simulink model "AirFlow"  (R2015a)
settings: Solver=ode45  StartTime=0.0  StopTime=10.0  RelTol=1e-3
settings Model: Creator=laragoxhaj  LastModifiedBy=laragoxhaj

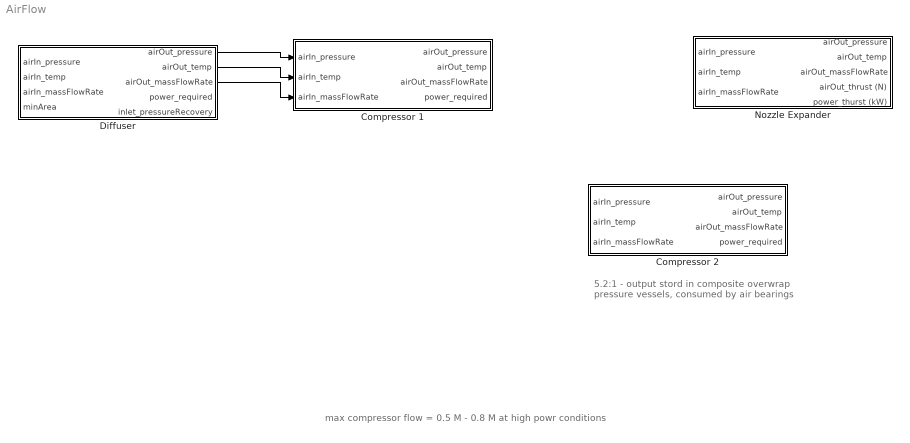
== system AirFlow ==
  note: max compressor flow = 0.5 M - 0.8 M at high powr conditions
  note: 5.2:1 - output stord in composite overwrap
      | pressure vessels, consumed by air bearings
  Compressor 1 : Subsystem
  Compressor 2 : Subsystem
  Diffuser : Subsystem
  Nozzle Expander : Subsystem
  wires:
  Diffuser/1(airOut_pressure) -> Compressor 1/1(airIn_pressure)
  Diffuser/2(airOut_temp) -> Compressor 1/2(airIn_temp)
  Diffuser/3(airOut_massFlowRate) -> Compressor 1/3(airIn_massFlowRate)

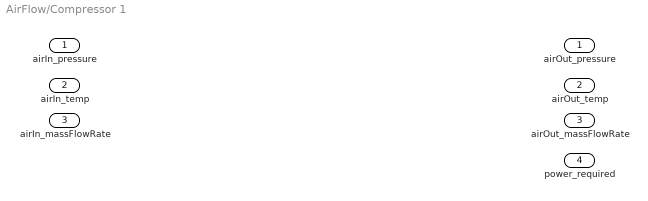
== system AirFlow/Compressor 1 ==
  airIn_pressure : Inport
  airIn_temp : Inport  Port=2
  airIn_massFlowRate : Inport  Port=3
  airOut_pressure : Outport
  airOut_temp : Outport  Port=2
  airOut_massFlowRate : Outport  Port=3
  power_required : Outport  Port=4

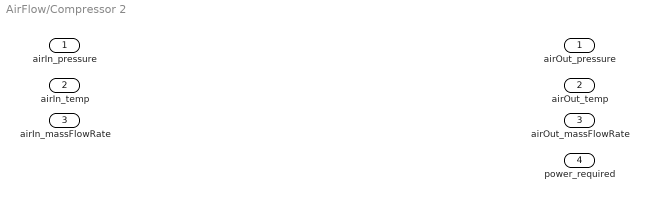
== system AirFlow/Compressor 2 ==
  airIn_pressure : Inport
  airIn_temp : Inport  Port=2
  airIn_massFlowRate : Inport  Port=3
  airOut_pressure : Outport
  airOut_temp : Outport  Port=2
  airOut_massFlowRate : Outport  Port=3
  power_required : Outport  Port=4

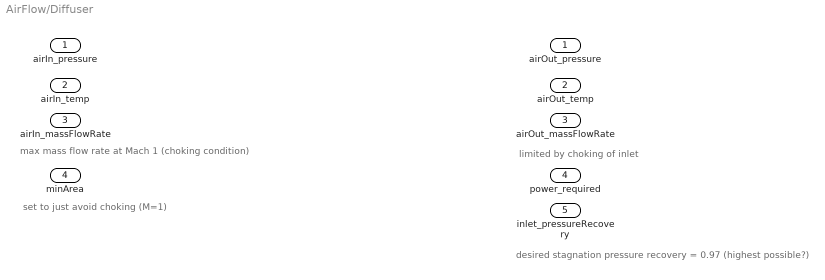
== system AirFlow/Diffuser ==
  note: set to just avoid choking (M=1)
  note: desired stagnation pressure recovery = 0.97 (highest possible?)
  note: limited by choking of inlet
  note: max mass flow rate at Mach 1 (choking condition)
  airIn_pressure : Inport
  airIn_temp : Inport  Port=2
  airIn_massFlowRate : Inport  Port=3
  minArea : Inport  Port=4
  airOut_pressure : Outport
  airOut_temp : Outport  Port=2
  airOut_massFlowRate : Outport  Port=3
  power_required : Outport  Port=4
  inlet_pressureRecovery : Outport  Port=5

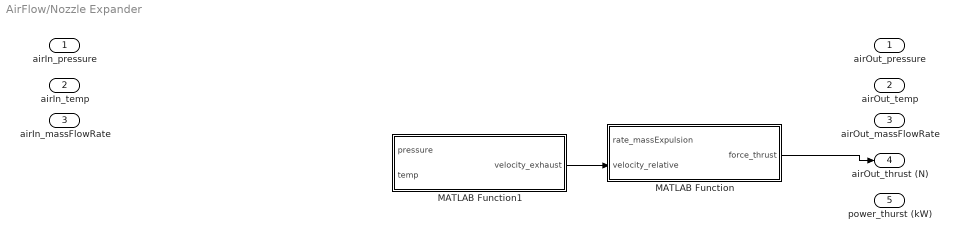
== system AirFlow/Nozzle Expander ==
  airIn_pressure : Inport
  airIn_temp : Inport  Port=2
  airIn_massFlowRate : Inport  Port=3
  MATLAB Function : MATLAB Function  TreatAsAtomicUnit=on
  MATLAB Function1 : MATLAB Function  TreatAsAtomicUnit=on
  airOut_pressure : Outport
  airOut_temp : Outport  Port=2
  airOut_massFlowRate : Outport  Port=3
  airOut_thrust (N) : Outport  Port=4
  power_thurst (kW) : Outport  Port=5
  wires:
  MATLAB Function/1(force_thrust) -> airOut_thrust (N)/1
  MATLAB Function1/1(velocity_exhaust) -> MATLAB Function/2(velocity_relative)

== matlab function AirFlow/Nozzle Expander/MATLAB Function1 ==
  data: pressure input; velocity_exhaust output; temp input
% m/s
function velocity_exhaust = fcn(pressure, temp)
velocity_exhaust = sqrt(2 * pressure * temp);

== matlab function AirFlow/Nozzle Expander/MATLAB Function ==
  data: rate_massExpulsion input; force_thrust output; velocity_relative input
% N
% rocket equation
function force_thrust = rocket_eqn(rate_massExpulsion, velocity_relative)
force_thrust = rate_massExpulsion, velocity_relative;
